simulink model "PX4_PID_HeadlessTrackingControllerVariableQuadDynamicsMdl"  (R2016b)
settings: Solver=FixedStepAuto  StartTime=0.0  StopTime=30  FixedStep=0.1  RelTol=1e-3  EnableMultiTasking=on
undefined symbols (not defined in the file): Params, QuaternionController_nav, TrackingWaypoint
libraries: pixhawk_slib_sensors_actuators x3, pixhawk_slib_uORB_RW x1
settings Model: Creator=Raj  LastModifiedBy=CDSLAB-User
settings DataIOCC: LimitDataPoints=on  SaveFormat=Array
settings OptimizationCC: LifeSpan=inf
settings DebuggingCC: UnderspecifiedInitializationDetection=Classic  MergeDetectMultiDrivingBlocksExec=none  SolverPrmCheckMsg=warning  StateNameClashWarn=warning  SFUnexpectedBacktrackingDiag=warning  SFNoUnconditionalDefaultTransitionDiag=warning  SFExecutionAtInitializationDiag=none
settings HardwareCC: ProdBitPerPointer=32  ProdBitPerSizeT=32  ProdBitPerPtrDiffT=32  ProdLargestAtomicFloat=None  ProdIntDivRoundTo=Undefined  ProdEndianess=Unspecified  ProdWordSize=32  ProdHWDeviceType=32-bit Generic
settings ModelReferenceCC: PropagateSignalLabelsOutOfModel=off
settings GRTTargetCC: TargetLangStandard=C89/C90 (ANSI)  GeneratePreprocessorConditionals=Disable all
settings ConfigComp: CovMetricSettings=dw  CovHtmlReporting=on  CovSaveCumulativeToWorkspaceVar=on  CovSaveSingleToWorkspaceVar=on  CovExternalEMLEnable=off  CovSFcnEnable=off

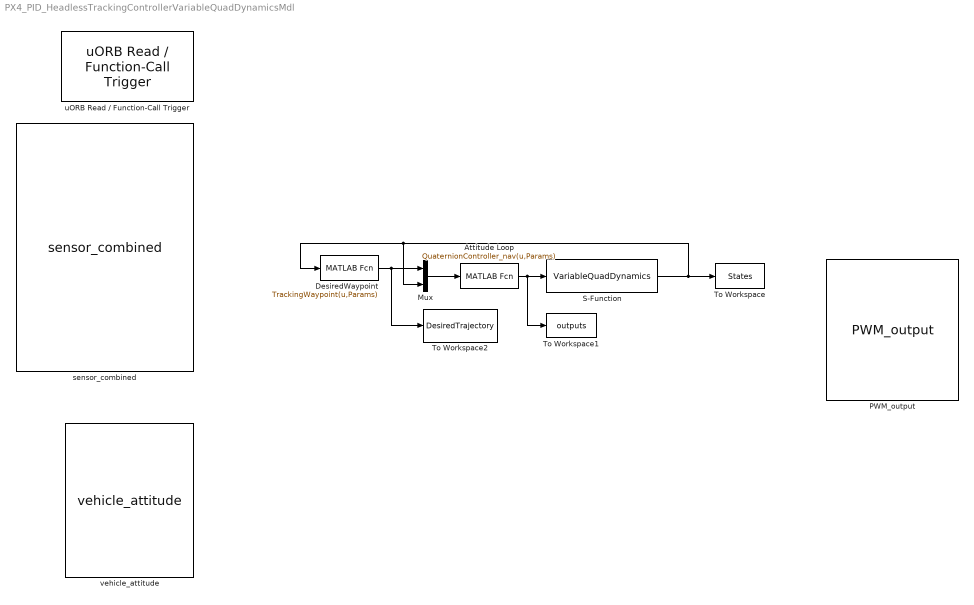
== system PX4_PID_HeadlessTrackingControllerVariableQuadDynamicsMdl ==
  Attitude Loop : MATLABFcn  MATLABFcn=QuaternionController_nav(u,Params)  OutputDimensions=4
  DesiredWaypoint : MATLABFcn  MATLABFcn=TrackingWaypoint(u,Params)  OutputDimensions=4
  Mux : Mux  Inputs=2
  PWM_output : pixhawk_slib_sensors_actuators/PWM_output  pwm_rate=400Hz  show_pwm1=on  show_pwm2=on  show_pwm3=on  show_pwm4=on  show_pwm5=off  show_pwm6=off  show_pwm7=off  show_pwm8=off
  S-Function : S-Function  FunctionName=VariableQuadDynamics  Parameters=Params  SFunctionDeploymentMode=off  EnableBusSupport=off
  To Workspace : ToWorkspace  VariableName=States  SaveFormat=Timeseries  SampleTime=-1
  To Workspace1 : ToWorkspace  VariableName=outputs  SaveFormat=Timeseries  SampleTime=-1
  To Workspace2 : ToWorkspace  VariableName=DesiredTrajectory  SaveFormat=Timeseries  SampleTime=-1
  sensor_combined : pixhawk_slib_sensors_actuators/sensor_combined  sampletime=1/250  show_mag=on  show_acc=on  show_gyro=on  show_baro=on  show_ts=on
  uORB Read / Function-Call Trigger : pixhawk_slib_uORB_RW/uORB Read // Function-Call Trigger  uORB_Topic_str='differential_pressure'  BusObjVar=Bus: differential_pressure_SL  uORB_Interval=1  AsyncOutput=on  Fcn_call_select=Generate Function Call Signal  TaskName='Task1'  Poll_timeout=100  Ts=-1
  vehicle_attitude : pixhawk_slib_sensors_actuators/vehicle_attitude  sampletime=1/250  show_r=on  show_p=on  show_y=on  show_q=on
  wires:
  Attitude Loop/1 -> S-Function/1, To Workspace1/1
  Mux/1 -> Attitude Loop/1
  DesiredWaypoint/1 -> Mux/1, To Workspace2/1
  S-Function/1 -> DesiredWaypoint/1, Mux/2, To Workspace/1
